simulink model "System_Loop_6"  (R2016b)
settings: Solver=FixedStepAuto  StartTime=0.0  StopTime=tF  FixedStep=0.01  RelTol=1e-3
values from neighbouring files (symbols this model uses):
  dt = 1e-7    (= 1e-07)    [parameters.m]
  flag = show_acc;  sim('System_Loop_6')    [Proj_6.m]
  K = K_r(i)    [Proj_1a.m]    (also in Proj_1b.m; Proj_5.m = K_i(i))
  K_dth = 0.05    [Proj_1b.m]    (also in Proj_5.m = -0.04; parameters.m = 0.05*sgn)
  M_d = M_d_r(i)    [Proj_7.m]    (also in parameters.m = 200*sgn)
  N = 3    [parameters.m]
  rho_u = mu(i)    [Proj_6.m]
  T_m = 120    [parameters.m]
  tau = tau_i(i)    [Proj_4.m]    (also in parameters.m = 0.05)
  tF = 1.5    [Controllers_Design.m]    (also in Proj_1a.m = 0.5; Proj_1b.m; Proj_2.m = 3; Proj_2_3.m = 5)
  Vc = 1250    [parameters.m]
  X_20 = dlambda*Vc*tF    [Proj_6.m]
settings Model: Creator=Daniel  LastModifiedBy=Daniel

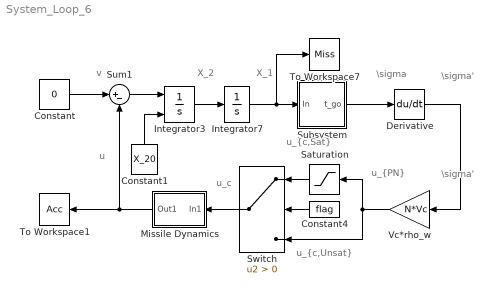
== system System_Loop_6 ==
  note: X_2
  note: v
  note: u_c
  note: u
  note: X_1
  note: \sigma
  note: \sigma'
  note: u_{PN}
  note: \sigma'
  note: u_{c,Unsat}
  note: u_{c,Sat}
  Constant : Constant  Value=0
  Constant1 : Constant  Value=X_20
      mask Display: image('X_20.PNG');
  Constant4 : Constant  Value=flag
  Derivative : Derivative
  Integrator3 : Integrator  InitialConditionSource=external
  Integrator7 : Integrator
  Missile Dynamics : Subsystem
      mask Display: image('Gm_s.PNG');
  Saturation : Saturate  UpperLimit=rho_u  LowerLimit=-rho_u
  Subsystem : Subsystem
      mask Display: image('t_go_Vc.png');
  Sum1 : Sum  Inputs=|+-
  Switch : Switch  Criteria=u2 > Threshold
  To Workspace1 : ToWorkspace  VariableName=Acc  SaveFormat=Timeseries  SampleTime=-1
  To Workspace7 : ToWorkspace  VariableName=Miss  SaveFormat=Timeseries  SampleTime=-1
  Vc*rho_w : Gain  Gain=N*Vc
  wires:
  Constant/1 -> Sum1/1
  Missile Dynamics/1(Out1) -> Sum1/2, To Workspace1/1
  Sum1/1 -> Integrator3/1
  Integrator3/1 -> Integrator7/1
  Subsystem/1(t_go) -> Derivative/1
  Switch/1 -> Missile Dynamics/1(In1)
  Derivative/1 -> Vc*rho_w/1
  Vc*rho_w/1 -> Switch/3, Saturation/1
  Constant1/1 -> Integrator3/2
  Integrator7/1 -> Subsystem/1(In), To Workspace7/1
  Constant4/1 -> Switch/2
  Saturation/1 -> Switch/1

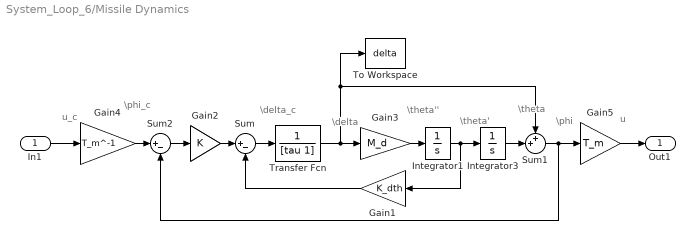
== system System_Loop_6/Missile Dynamics ==
  note: \theta'
  note: \theta''
  note: \theta
  note: \delta
  note: \delta_c
  note: \phi_c
  note: \phi
  note: u
  note: u_c
  In1 : Inport
  Gain1 : Gain  Gain=K_dth
  Gain2 : Gain  Gain=K
  Gain3 : Gain  Gain=M_d
  Gain4 : Gain  Gain=T_m^-1
  Gain5 : Gain  Gain=T_m
  Integrator1 : Integrator
  Integrator3 : Integrator
  Sum : Sum  Inputs=|+-
  Sum1 : Sum  Inputs=++|
  Sum2 : Sum  Inputs=|+-
  To Workspace : ToWorkspace  VariableName=delta  SaveFormat=Timeseries  SampleTime=-1
  Transfer Fcn : TransferFcn  Denominator=[tau 1]
  Out1 : Outport
  wires:
  Gain1/1 -> Sum/2
  Sum/1 -> Transfer Fcn/1
  Gain2/1 -> Sum/1
  Sum1/1 -> Sum2/2, Gain5/1
  Gain3/1 -> Integrator1/1
  Integrator1/1 -> Integrator3/1, Gain1/1
  Integrator3/1 -> Sum1/2
  Sum2/1 -> Gain2/1
  Gain5/1 -> Out1/1
  In1/1 -> Gain4/1
  Gain4/1 -> Sum2/1
  Transfer Fcn/1 -> Sum1/1, To Workspace/1, Gain3/1

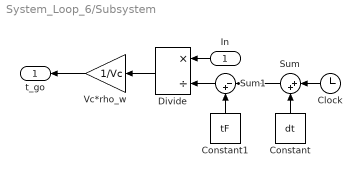
== system System_Loop_6/Subsystem ==
  In : Inport
  Clock : Clock
  Constant : Constant  Value=dt
  Constant1 : Constant  Value=tF
  Divide : Product  Inputs=*/
  Sum : Sum  Inputs=|++
  Sum1 : Sum  Inputs=|-+
  Vc*rho_w : Gain  Gain=1/Vc
  t_go : Outport
  wires:
  Sum/1 -> Sum1/1
  In/1 -> Divide/1
  Divide/1 -> Vc*rho_w/1
  Constant/1 -> Sum/2
  Clock/1 -> Sum/1
  Vc*rho_w/1 -> t_go/1
  Sum1/1 -> Divide/2
  Constant1/1 -> Sum1/2
